simulink model "basic_pid_torque"  (R2015a)
settings: Solver=ode45  StartTime=0.0  StopTime=10.0  RelTol=1e-3
values from neighbouring files (symbols this model uses):
  k_s = i    [multi_pass.m]    (also in parameters.m = 120)
  pid_torque_Kd = 0    [parameters.m]
  pid_torque_Ki = 1    [parameters.m]
  pid_torque_Kp = 0.1    [parameters.m]
  tau_max = 5    [parameters.m]
undefined symbols (not defined in the file or in its folder): fdesignblkfcn, gcbh, pid
libraries: simulink x1, dsparch4 x1
settings Model: Creator=preston  LastModifiedBy=Nathan

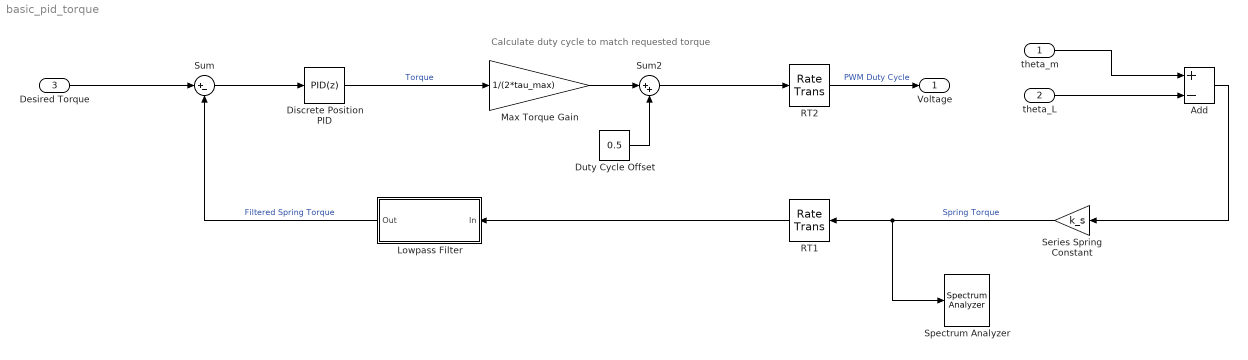
== system basic_pid_torque ==
  note: Calculate duty cycle to match requested torque
  theta_m : Inport
  theta_L : Inport  Port=2
  Desired Torque : Inport  Port=3
  Add : Sum  Inputs=+-
  Discrete Position PID : simulink/Continuous/PID Controller  Controller=PID  TimeDomain=Discrete-time  SampleTime=-1  IntegratorMethod=Backward Euler  FilterMethod=Forward Euler  Form=Parallel  UseFilter=off  ControllerParametersSource=internal  P=pid_torque_Kp  I=pid_torque_Ki  D=pid_torque_Kd  N=pid.N  InitialConditionSource=internal  InitialConditionForIntegrator=0  InitialConditionForFilter=0  ExternalReset=none  LimitOutput=on  UpperSaturationLimit=tau_max  LowerSaturationLimit=-tau_max  LinearizeAsGain=off  AntiWindupMode=none  Kb=1  TrackingMode=off  Kt=1  PParamMin=[]  PParamMax=[]  IParamMin=[]  IParamMax=[]  DParamMin=[]  DParamMax=[]  NParamMin=[]  NParamMax=[]  KbParamMin=[]  KbParamMax=[]  KtParamMin=[]  KtParamMax=[]  POutMin=[]  POutMax=[]  IOutMin=[]  IOutMax=[]  DOutMin=[]  DOutMax=[]  NOutMin=[]  NOutMax=[]  KbOutMin=[]  KbOutMax=[]  KtOutMin=[]  KtOutMax=[]  IntegratorOutMin=[]  IntegratorOutMax=[]  FilterOutMin=[]  FilterOutMax=[]  SumOutMin=[]  SumOutMax=[]  SumI1OutMin=[]  SumI1OutMax=[]  SumI2OutMin=[]  SumI2OutMax=[]  SumI3OutMin=[]  SumI3OutMax=[]  SumDOutMin=[]  SumDOutMax=[]  SaturationOutMin=[]  SaturationOutMax=[]  IntegratorContinuousStateAttributes=''  IntegratorStateMustResolveToSignalObject=off  IntegratorRTWStateStorageClass=Auto  FilterContinuousStateAttributes=''  FilterStateMustResolveToSignalObject=off  FilterRTWStateStorageClass=Auto  DifferentiatorICPrevScaledInput=0  DifferentiatorOutMin=[]  DifferentiatorOutMax=[]
  Duty Cycle Offset : Constant  Value=0.5
  Lowpass Filter : Subsystem  DialogController=fdesignblkfcn  InitFcn=fdesignblkfcn(gcbh, {'InitFcn'});  mask(Lowpass Filter){}
      mask help: Design a lowpass filter
      settings: CopyFcn=fdesignblkfcn(gcbh, {'CopyFcn'});
      mask Help: helpview(mapfilelocation('dsp'), 'dsplowpassfilter');
      mask Display: disp('Lowpass')
  Max Torque Gain : Gain  Gain=1/(2*tau_max)
  RT1 : RateTransition  OutPortSampleTime=T_sample_control
  RT2 : RateTransition
  Series Spring Constant : Gain  Gain=k_s
  Spectrum Analyzer : SpectrumAnalyzer
  Sum : Sum  Inputs=|+-
  Sum2 : Sum  Inputs=|++
  Voltage : Outport
  wires:
  RT2/1 -> Voltage/1  "PWM Duty Cycle"
  Sum/1 -> Discrete Position PID/1
  Series Spring Constant/1 -> Spectrum Analyzer/1, RT1/1  "Spring Torque"
  Add/1 -> Series Spring Constant/1
  RT1/1 -> Lowpass Filter/1(In)
  theta_m/1 -> Add/1
  theta_L/1 -> Add/2
  Desired Torque/1 -> Sum/1
  Discrete Position PID/1 -> Max Torque Gain/1  "Torque"
  Max Torque Gain/1 -> Sum2/1
  Sum2/1 -> RT2/1
  Duty Cycle Offset/1 -> Sum2/2
  Lowpass Filter/1(Out) -> Sum/2  "Filtered Spring Torque"

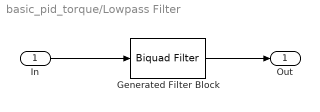
== system basic_pid_torque/Lowpass Filter ==
  In : Inport
  Generated Filter Block : dsparch4/Biquad Filter  Tag=BlockMethodSubSystem  IIRFiltStruct=Direct form II  CoeffSource=Specify via dialog  BiQuadCoeffs=[0.25000019876766189 0.50000039753532377 0.25000019876766189 1 -1.899333420104083 0.90416304086512334]  a0Flag=Warning  IC=0  ICnum=0  ICden=0  InputProcessing=Columns as channels (frame based)  denAccumFracLength=30  denProdOutputFracLength=30  secondMemoryFracLength=15  roundingMode=Floor  overflowMode=off  ScaleValues=[0.0048296169211536049;1]  optimizeScaleValues=off  ScaleValueMode=Specify via input port (g)  scaleValueFracLength=14  FilterSource=Specify via dialog  FilterObject=Hm_biquad
  Out : Outport
  wires:
  In/1 -> Generated Filter Block/1
  Generated Filter Block/1 -> Out/1
